simulink model "AFS_sim"  (R2023a)
settings: Solver=FixedStepAuto  StartTime=0.0  StopTime=Tf  RelTol=1e-2
values from neighbouring files (symbols this model uses):
  vehicle_data = getVehicleDataStruct()    [main.m]
undefined symbols (not defined in the file or in its folder): input
libraries: autolibshared x1
settings Model: Creator=ashkan  LastModifiedBy=ashkan
settings OptimizationCC: ReuseModelBlockBuffer=off

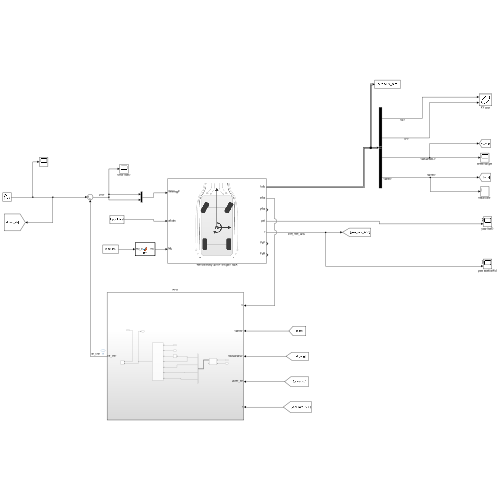
[thumbnail: Simulink's stored preview of the top-level diagram]
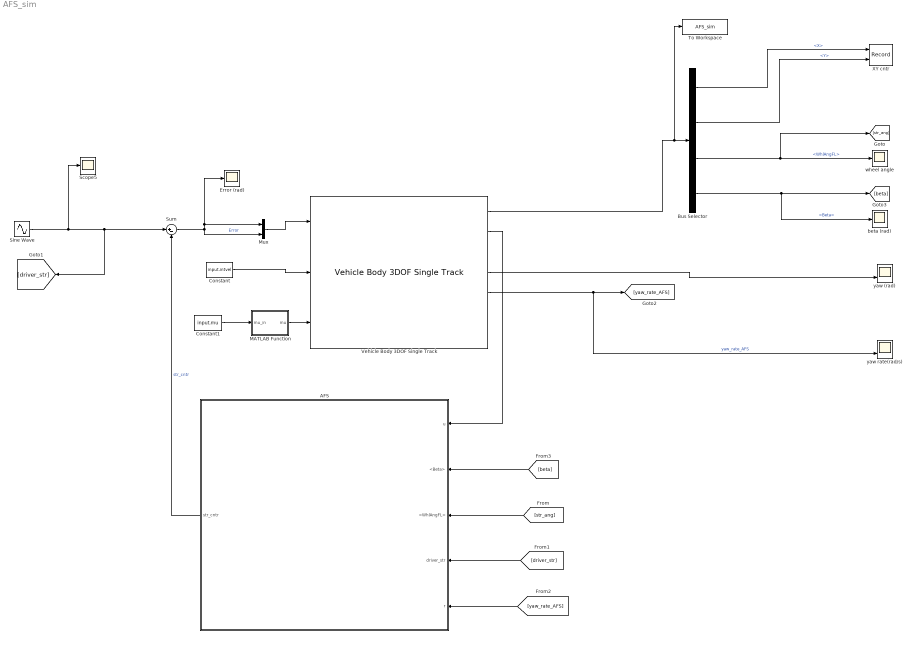
== system AFS_sim ==
  AFS : Subsystem
  Bus Selector : BusSelector  OutputSignals=InertFrm.Cg.Disp.X,InertFrm.Cg.Disp.Y,BdyFrm.FrntAxl.Steer.WhlAngFL,BdyFrm.Cg.Ang.Beta
  Constant : Constant  Value=input.intvel
  Constant1 : Constant  Value=input.mu
  Error (rad) : Scope
  MATLAB Function : MATLAB Function  TreatAsAtomicUnit=on
  Mux : Mux  Inputs=2
  Scope5 : Scope
  Sine Wave : Sin  Amplitude=input.str.amp  Frequency=input.str.freq  SampleTime=input.str.sample_time
  Sum : Sum  Inputs=|+-
  To Workspace : ToWorkspace  VariableName=AFS_sim  SaveFormat=Timeseries  SampleTime=-1
  Vehicle Body 3DOF Single Track : autolibshared/Vehicle Body 3DOF Single Track  trackMode=Dual  inputMode=External longitudinal velocity  frontSteerMode=on  rearSteerMode=off  windMode=off  muMode=on  extFMode=off  extMMode=off  htchFMode=off  htchMMode=off  extXo=off  extpsio=off  extxdoto=off  extro=off  extYo=off  extTamb=off  extydoto=off  aMode=2  NF=2  NR=2  m=vehicle_data.vehicle.m  a=vehicle_data.vehicle.Lf  b=vehicle_data.vehicle.Lr  h=vehicle_data.vehicle.hGs  dh=1  hh=0.2  X_o=0  xdot_o=0  CalphaMode=off  sigmaMode=off  d=0  hl=0  w="[vehicle_data.vehicle.Wf ,  vehicle_data.vehicle.Wr]"  Cy_f=vehicle_data.front_suspension.Ks_f  Cy_r=vehicle_data.rear_suspension.Ks_r  sigma_f=.1  sigma_r=.1  alpha_f_brk=[-.1 .1]  Cy_f_data=[-9e3 9e3]  alpha_r_brk=[-.1 .1]  Cy_r_data=[-9e3 9e3]  Y_o=0  ydot_o=0  Izz=4000  psi_o=0  r_o=0  Af=2  Cd=.3  Cl=.1  Cpm=.1  beta_w=[0 0.01:0.01:0.3]  Cs=[0 0.01:0.01:0.3]  Cym=[0 1e-6:0.01:0.3]  Pabs=101325  Tair=273  g=9.81  mu=1  xdot_tol=.01  Fznom=5000  Fxtire_sat=7e4  Fytire_sat=7e4  longOff=0  latOff=0  vertOff=0  wrapAng=off
  XY cntr : Record  FileSettingsInternal="{\"entries\":[{\"content\":{\"excelSettings\":{\"content\":{},\"type\":\"Streamout.ExcelSettings\"}},\"type\":\"Streamout.FileSettingStorage\",\"uuid\":\"\"}],\"packageUris\":[\"http:\\/\\/schema.mathworks.com\\/mf0\\/streamout_blocks\\/R2020a\"],\"version\":\"1.0\"}"  Layout=[1 1]  SignalsInternal="{\"entries\":[{\"content\":{\"signals\":[{\"content\":{\"blockPath\":[],\"dimensions\":[1],\"domain\":\"\",\"lineColor\":\"#22b573\",\"plots\":[1],\"port\":1,\"sid\":[\"\"],\"signalID\":28844,\"signalName\":\"<X>\"},\"type\":\"RecordBlkView.Signal\",\"uuid\":\"\"},{\"content\":{\"blockPath\":[],\"dimensions\":[1],\"domain\":\"\",\"lineColor\":\"#0072bd\",\"plots\":[1],\"port\":2,\"sid\":[\"\"],\"signalID\":28848,\"signalName\":\"<Y>\"},\"type\":\"RecordBlkView.Signal\",\"uuid\":\"\"}]},\"type\":\"RecordBlkView.InputSignals\",\"uuid\":\"\"}],\"packageUris\":[\"http:\\/\\/schema.mathworks.com\\/mf0\\/streamout_blocks\\/R2020a\"],\"version\":\"1.0\"}"  VisualizationBindings="{\"xyplotplugin\":{\"info\":[{\"series\":[{\"bindingParametersList\":[{\"parameter\":\"X-Axis\",\"signalID\":28844,\"signalName\":\"<X>\"},{\"parameter\":\"Y-Axis\",\"signalID\":28848,\"signalName\":\"<Y>\"}],\"seriesID\":17755}],\"subplotID\":1}]}}"  CompatibilityTag=XY
  beta (rad) : Scope
  wheel angle : Scope
  yaw (rad) : Scope  NumInputPorts=2
  yaw rate(rad/s) : Scope  NumInputPorts=2
  wires:
  Bus Selector/3 -> [str_ang], wheel angle/1  "<WhlAngFL>"
  Bus Selector/1 -> XY cntr/1  "<X>"
  Bus Selector/2 -> XY cntr/2  "<Y>"
  Sum/1 -> Mux/2, Mux/1, Error (rad)/1  "Error"
  Bus Selector/4 -> [beta], beta (rad)/1  "<Beta>"
  Sine Wave/1 -> [driver_str], Sum/1, Scope5/1
  Vehicle Body 3DOF Single Track/1 -> To Workspace/1, Bus Selector/1
  Vehicle Body 3DOF Single Track/5 -> [yaw_rate_AFS], yaw rate(rad/s)/2  "yaw_rate_AFS"
  Constant/1 -> Vehicle Body 3DOF Single Track/2
  Vehicle Body 3DOF Single Track/4 -> yaw (rad)/2
  Vehicle Body 3DOF Single Track/2 -> AFS/1(u)
  AFS/1(str_cntr) -> Sum/2  "str_cntr"
  [str_ang] -> AFS/3(<WhlAngFL>)
  [driver_str] -> AFS/4(driver_str)
  [yaw_rate_AFS] -> AFS/5(r)
  [beta] -> AFS/2(<Beta>)
  Mux/1 -> Vehicle Body 3DOF Single Track/1
  MATLAB Function/1(mu) -> Vehicle Body 3DOF Single Track/3
  Constant1/1 -> MATLAB Function/1(mu_in)

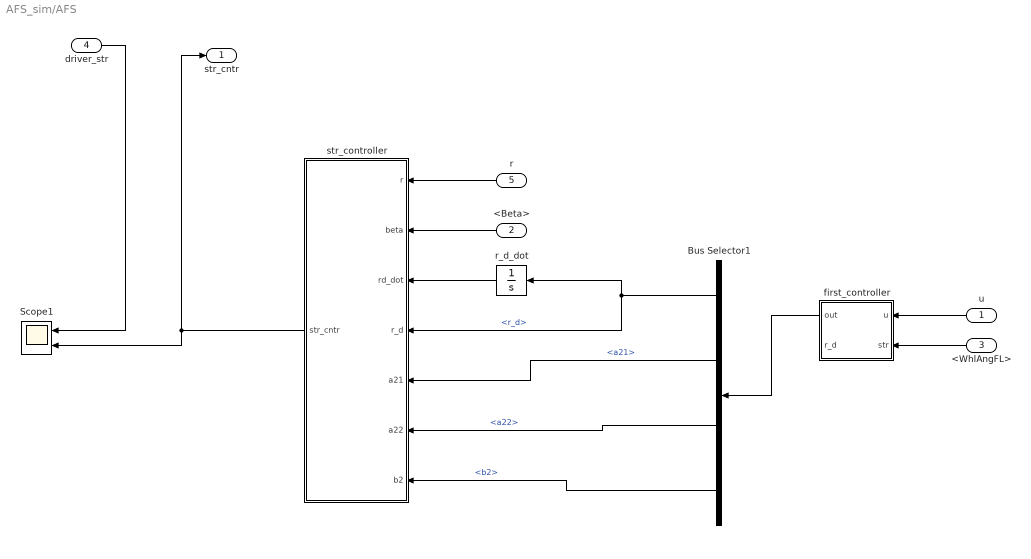
== system AFS_sim/AFS ==
  u : Inport
  <Beta> : Inport  Port=2
  <WhlAngFL> : Inport  Port=3
  driver_str : Inport  Port=4
  r : Inport  Port=5
  Bus Selector1 : BusSelector  OutputSignals=r_d,a21,a22,b2
  Scope1 : Scope  NumInputPorts=2
  first_controller : MATLAB Function  TreatAsAtomicUnit=on
  r_d_dot : Integrator
  str_controller : MATLAB Function  TreatAsAtomicUnit=on
  str_cntr : Outport
  wires:
  driver_str/1 -> Scope1/1
  <Beta>/1 -> str_controller/2(beta)
  r/1 -> str_controller/1(r)
  first_controller/1(out) -> Bus Selector1/1
  <WhlAngFL>/1 -> first_controller/2(str)
  u/1 -> first_controller/1(u)
  Bus Selector1/2 -> str_controller/5(a21)  "<a21>"
  Bus Selector1/3 -> str_controller/6(a22)  "<a22>"
  str_controller/1(str_cntr) -> str_cntr/1, Scope1/2
  r_d_dot/1 -> str_controller/3(rd_dot)
  Bus Selector1/1 -> str_controller/4(r_d), r_d_dot/1  "<r_d>"
  Bus Selector1/4 -> str_controller/7(b2)  "<b2>"

== matlab function AFS_sim/AFS/str_controller ==
  data: r input; beta input; rd_dot input; r_d input; a21 input; str_cntr output; a22 input; b2 input; vehicle_data parameter
function str_cntr = str_controller(r, beta , rd_dot , r_d , a21 , a22 , b2, vehicle_data)

%    lambda = AFS.lambda;
    s = r - r_d;
    lambda = vehicle_data.AFS.lambda;
    X      = vehicle_data.AFS.X;
    str_cntr = ((1/b2) * (-a21*beta - a22*r + rd_dot - lambda*(s))) - sign(s)*X;


end

== matlab function AFS_sim/AFS/first_controller ==
  data: out output Bus: out_rd_bus; u input; str input; vehicle_data parameter; r_d output
function [out, r_d] = r_d(u , str, vehicle_data)


% here is some simplified parameters :)
   m = vehicle_data.vehicle.m;
   a = vehicle_data.vehicle.Lf;
   b = vehicle_data.vehicle.Lr;
   izz = vehicle_data.vehicle.i_zz;
   g = vehicle_data.vehicle.g;
   L = vehicle_data.vehicle.L;
   mu = vehicle_data.AFS.mu;  % --> should come from scenario
   Caf = vehicle_data.front_suspension.Ks_f ;
   Car = vehicle_data.rear_suspension.Ks_r;
   
   
% lets calculate some live parameters!!! _|_
    
   r_up_lim = 0.85 * abs(mu*g / u);
   r_ss = (2*L*Caf*Car*u)/(2*Car*Caf*L^2 - m*u^2*(a*Caf - b*Car)) * str;
   r_d = min(r_ss , r_up_lim)* sign(str);
 
   a11 = (-2*Caf - 2*Car)/(m * u);
   a12 = -1 + (2*Car*b - 2*Caf*a)/(m * u^2);
   a21 = (2*Car*b - 2*Caf*a)/izz;
   a22 = (-2*Caf*a^2 - 2*Car*b^2)/(izz * u);
   b1 = (2*Caf)/(m * u);
   b2 = (2 * Caf * a)/izz;

% outputs
   out.a11 = a11;
   out.a21 = a21;
   out.a12 = a12;
   out.a22 = a22;
   out.b1 = b1;
   out.b2 = b2;
   out.r_d = r_d;

end

== matlab function AFS_sim/MATLAB Function ==
  data: mu_in input; mu output
function mu = fcn(mu_in)

mu = mu_in*ones(2);
